simulink model "Throttle_and_UI_Module"  (R2025a)
settings: Solver=VariableStepAuto
settings Model: Creator=MSII  LastModifiedBy=ASUS

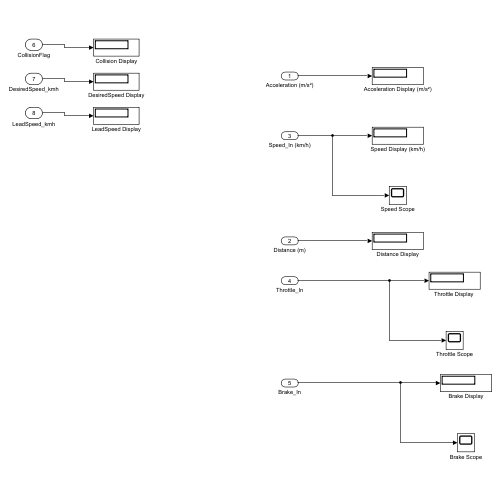
[thumbnail: Simulink's stored preview of the top-level diagram]
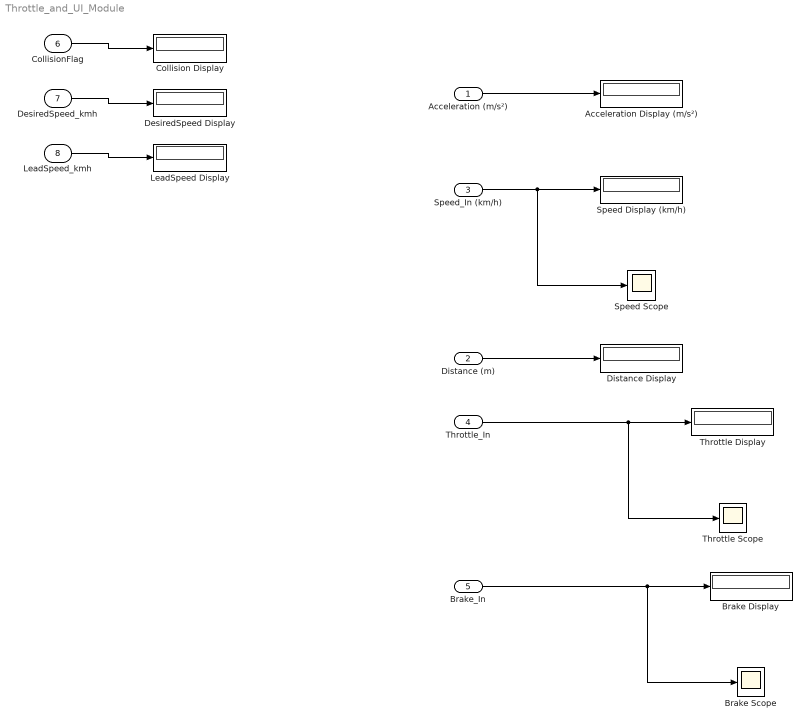
== system Throttle_and_UI_Module ==
  Acceleration (m/s²) : Inport
  Distance (m) : Inport  Port=2
  Speed_In (km/h) : Inport  Port=3
  Throttle_In : Inport  Port=4
  Brake_In : Inport  Port=5
  CollisionFlag : Inport  Port=6  OutDataTypeStr=boolean
  DesiredSpeed_kmh : Inport  Port=7
  LeadSpeed_kmh : Inport  Port=8
  Acceleration Display (m/s²) : Display
  Brake Display : Display
  Brake Scope : Scope
      settings: ActiveDisplayYMinimum=-82.044400764956549  ActiveDisplayYMaximum=157.51047775665415  DataLoggingVariableName=ScopeData2
  Collision Display : Display
  DesiredSpeed Display : Display
  Distance Display : Display
  LeadSpeed Display : Display
  Speed Display (km/h) : Display
  Speed Scope : Scope
      settings: ActiveDisplayYMinimum=-126.42503132575258  ActiveDisplayYMaximum=137.68422224432354
  "Throttle Display " : Display
  Throttle Scope : Scope
      settings: ActiveDisplayYMinimum=-48.82668692343433  ActiveDisplayYMaximum=113.31348422599231
  wires:
  Speed_In (km/h)/1 -> Speed Scope/1, Speed Display (km/h)/1
  Distance (m)/1 -> Distance Display/1
  Acceleration (m/s²)/1 -> Acceleration Display (m/s²)/1
  Throttle_In/1 -> Throttle Scope/1, "Throttle Display "/1
  Brake_In/1 -> Brake Scope/1, Brake Display/1
  CollisionFlag/1 -> Collision Display/1
  DesiredSpeed_kmh/1 -> DesiredSpeed Display/1
  LeadSpeed_kmh/1 -> LeadSpeed Display/1
